simulink model "Regulacia_JCBM_Uloha3_S"  (R2022b)
settings: Solver=VariableStepAuto  StartTime=0.0  StopTime=4  RelTol=1e-8
values from neighbouring files (symbols this model uses):
  cfi = (Ua-Ra*IN)/wN    (= 2.66063720525)    [Regulacia_JCBM_M.m]
  h1 = double(h(1))    [Regulacia_JCBM_M.m]
  h2 = double(h(2))    [Regulacia_JCBM_M.m]
  Jc = Jm*8    (= 2.32)    [Regulacia_JCBM_M.m]
  Ki_2 = double(Ki_2)    [Regulacia_JCBM_M.m]
  Ki_5 = double(Ki_5)    [Regulacia_JCBM_M.m]
  La = 0.0081    [Regulacia_JCBM_M.m]
  Mz = MN    (= 132)    [Regulacia_JCBM_M.m]
  r1_2 = double(r1_2)    [Regulacia_JCBM_M.m]
  r1_5 = double(r1_5)    [Regulacia_JCBM_M.m]
  r2_2 = double(r2_2)    [Regulacia_JCBM_M.m]
  r2_5 = double(r2_5)    [Regulacia_JCBM_M.m]
  Ra = 0.522    [Regulacia_JCBM_M.m]
settings Model: Creator=hwswi  LastModifiedBy=hwswi

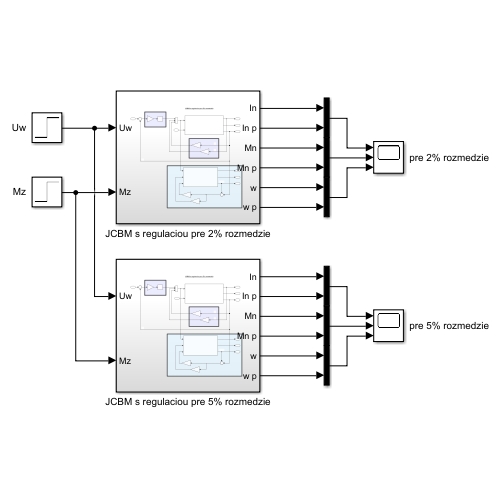
[thumbnail: Simulink's stored preview of the top-level diagram]
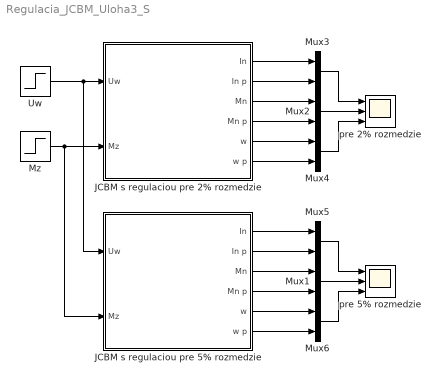
== system Regulacia_JCBM_Uloha3_S ==
  JCBM s regulaciou pre 2% rozmedzie : Subsystem
  JCBM s regulaciou pre 5% rozmedzie : Subsystem
  Mux{1..6} (6 alike) : Mux  Inputs=2
  Mz : Step  Time=2  After=Mz  SampleTime=0
  Uw : Step  Time=0  After=100  SampleTime=0
  pre 2% rozmedzie : Scope  NumInputPorts=3
  pre 5% rozmedzie : Scope  NumInputPorts=3
  wires:
  Uw/1 -> JCBM s regulaciou pre 5% rozmedzie/1(Uw), JCBM s regulaciou pre 2% rozmedzie/1(Uw)
  JCBM s regulaciou pre 2% rozmedzie/1(In) -> Mux3/1
  JCBM s regulaciou pre 2% rozmedzie/2(In p) -> Mux3/2
  JCBM s regulaciou pre 2% rozmedzie/4(Mn p) -> Mux2/2
  JCBM s regulaciou pre 2% rozmedzie/3(Mn) -> Mux2/1
  JCBM s regulaciou pre 2% rozmedzie/6(w p) -> Mux4/2
  JCBM s regulaciou pre 2% rozmedzie/5(w) -> Mux4/1
  JCBM s regulaciou pre 5% rozmedzie/5(w) -> Mux6/1
  JCBM s regulaciou pre 5% rozmedzie/6(w p) -> Mux6/2
  JCBM s regulaciou pre 5% rozmedzie/3(Mn) -> Mux1/1
  JCBM s regulaciou pre 5% rozmedzie/4(Mn p) -> Mux1/2
  JCBM s regulaciou pre 5% rozmedzie/2(In p) -> Mux5/2
  JCBM s regulaciou pre 5% rozmedzie/1(In) -> Mux5/1
  Mux4/1 -> pre 2% rozmedzie/3
  Mux6/1 -> pre 5% rozmedzie/3
  Mux2/1 -> pre 2% rozmedzie/2
  Mux1/1 -> pre 5% rozmedzie/2
  Mux5/1 -> pre 5% rozmedzie/1
  Mux3/1 -> pre 2% rozmedzie/1
  Mz/1 -> JCBM s regulaciou pre 5% rozmedzie/2(Mz), JCBM s regulaciou pre 2% rozmedzie/2(Mz)

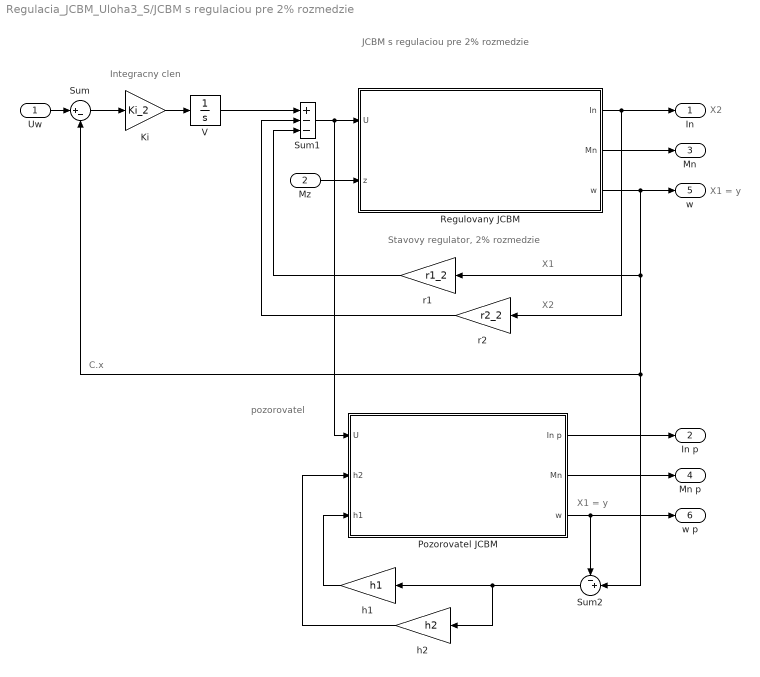
== system Regulacia_JCBM_Uloha3_S/JCBM s regulaciou pre 2% rozmedzie ==
  note: pozorovatel
  note: X1 = y
  note: X1 = y
  note: Stavovy regulator, 2% rozmedzie
  note: X2
  note: X1
  note: JCBM s regulaciou pre 2% rozmedzie
  note: Integracny clen
  note: X2
  note: C.x
  Uw : Inport
  Mz : Inport  Port=2
  Ki : Gain  Gain=Ki_2
  Pozorovatel JCBM : Subsystem
  Regulovany JCBM : Subsystem
  Sum : Sum  Inputs=|+-
  Sum1 : Sum  Inputs=+--
  Sum2 : Sum  Inputs=-+|
  V : Integrator
  h1 : Gain  Gain=h1
  h2 : Gain  Gain=h2
  "r1 " : Gain  Gain=r1_2
  "r2 " : Gain  Gain=r2_2
  In : Outport
  In p : Outport  Port=2
  Mn : Outport  Port=3
  Mn p : Outport  Port=4
  w : Outport  Port=5
  w p : Outport  Port=6
  wires:
  Uw/1 -> Sum/1
  Pozorovatel JCBM/3(w) -> w p/1, Sum2/1
  "r1 "/1 -> Sum1/3
  Sum1/1 -> Pozorovatel JCBM/1(U), Regulovany JCBM/1(U)
  Sum2/1 -> h2/1, h1/1
  Regulovany JCBM/1(In) -> "r2 "/1, In/1
  Regulovany JCBM/3(w) -> w/1, Sum2/2, Sum/2, "r1 "/1
  Ki/1 -> V/1
  "r2 "/1 -> Sum1/2
  Sum/1 -> Ki/1
  V/1 -> Sum1/1
  h2/1 -> Pozorovatel JCBM/2(h2)
  h1/1 -> Pozorovatel JCBM/3(h1)
  Regulovany JCBM/2(Mn) -> Mn/1
  Pozorovatel JCBM/1(In p) -> In p/1
  Pozorovatel JCBM/2(Mn) -> Mn p/1
  Mz/1 -> Regulovany JCBM/2(z)

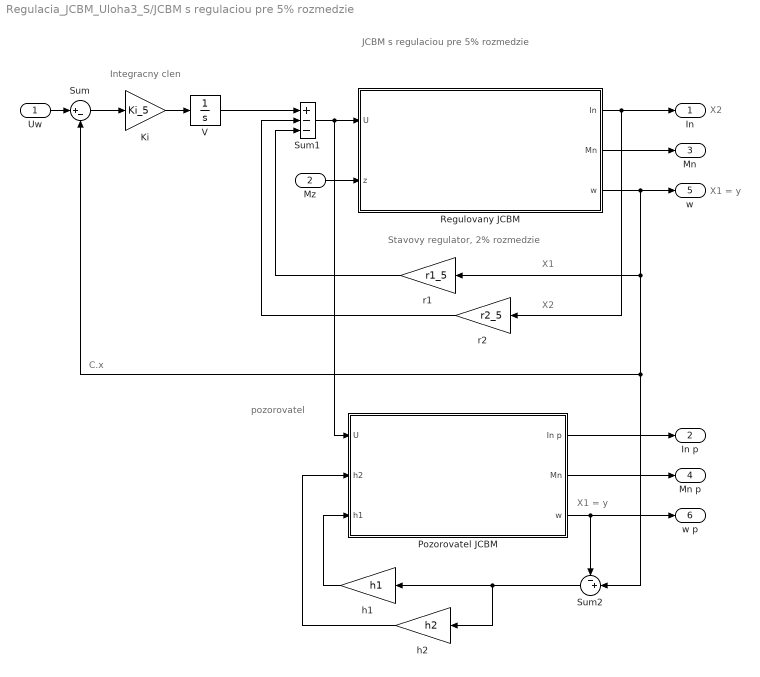
== system Regulacia_JCBM_Uloha3_S/JCBM s regulaciou pre 5% rozmedzie ==
  note: X1 = y
  note: pozorovatel
  note: X1
  note: Integracny clen
  note: JCBM s regulaciou pre 5% rozmedzie
  note: Stavovy regulator, 2% rozmedzie
  note: X2
  note: X2
  note: X1 = y
  note: C.x
  Uw : Inport
  Mz : Inport  Port=2
  Ki : Gain  Gain=Ki_5
  Pozorovatel JCBM : Subsystem
  Regulovany JCBM : Subsystem
  Sum : Sum  Inputs=|+-
  Sum1 : Sum  Inputs=+--
  Sum2 : Sum  Inputs=-+|
  V : Integrator
  h1 : Gain  Gain=h1
  h2 : Gain  Gain=h2
  "r1 " : Gain  Gain=r1_5
  "r2 " : Gain  Gain=r2_5
  In : Outport
  In p : Outport  Port=2
  Mn : Outport  Port=3
  Mn p : Outport  Port=4
  w : Outport  Port=5
  w p : Outport  Port=6
  wires:
  Regulovany JCBM/3(w) -> w/1, Sum2/2, Sum/2, "r1 "/1
  Regulovany JCBM/2(Mn) -> Mn/1
  "r1 "/1 -> Sum1/3
  V/1 -> Sum1/1
  Pozorovatel JCBM/1(In p) -> In p/1
  "r2 "/1 -> Sum1/2
  Ki/1 -> V/1
  Sum1/1 -> Pozorovatel JCBM/1(U), Regulovany JCBM/1(U)
  h2/1 -> Pozorovatel JCBM/2(h2)
  Pozorovatel JCBM/3(w) -> w p/1, Sum2/1
  Pozorovatel JCBM/2(Mn) -> Mn p/1
  h1/1 -> Pozorovatel JCBM/3(h1)
  Sum2/1 -> h2/1, h1/1
  Regulovany JCBM/1(In) -> "r2 "/1, In/1
  Sum/1 -> Ki/1
  Uw/1 -> Sum/1
  Mz/1 -> Regulovany JCBM/2(z)

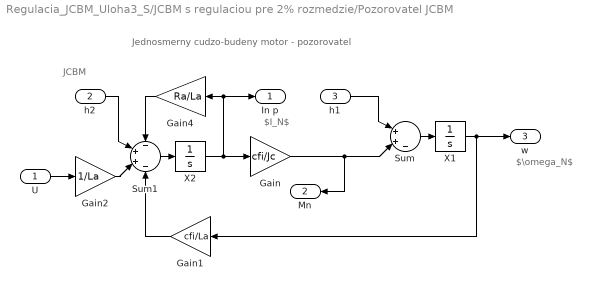
== system Regulacia_JCBM_Uloha3_S/JCBM s regulaciou pre 2% rozmedzie/Pozorovatel JCBM ==
  note: JCBM
  note: Jednosmerny cudzo-budeny motor - pozorovatel
  note: $\omega_N$
  note: $I_N$
  U : Inport
  h2 : Inport  Port=2
  h1 : Inport  Port=3
  Gain : Gain  Gain=cfi/Jc
  Gain1 : Gain  Gain=cfi/La
  Gain2 : Gain  Gain=1/La
  Gain4 : Gain  Gain=Ra/La
  Sum : Sum  Inputs=|++-
  Sum1 : Sum  Inputs=-++-
  X1 : Integrator
  X2 : Integrator
  In p : Outport
  Mn : Outport  Port=2
  w : Outport  Port=3
  wires:
  X1/1 -> Gain1/1, w/1
  X2/1 -> Gain/1, In p/1, Gain4/1
  Gain4/1 -> Sum1/1
  Sum1/1 -> X2/1
  Gain1/1 -> Sum1/4
  Sum/1 -> X1/1
  Gain2/1 -> Sum1/3
  U/1 -> Gain2/1
  h1/1 -> Sum/1
  h2/1 -> Sum1/2
  Gain/1 -> Mn/1, Sum/2

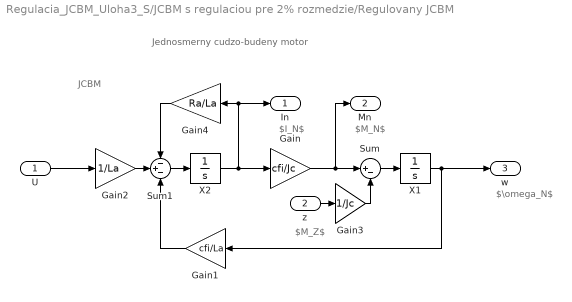
== system Regulacia_JCBM_Uloha3_S/JCBM s regulaciou pre 2% rozmedzie/Regulovany JCBM ==
  note: $M_N$
  note: $I_N$
  note: $\omega_N$
  note: Jednosmerny cudzo-budeny motor
  note: JCBM
  note: $M_Z$
  U : Inport
  z : Inport  Port=2
  Gain : Gain  Gain=cfi/Jc
  Gain1 : Gain  Gain=cfi/La
  Gain2 : Gain  Gain=1/La
  Gain3 : Gain  Gain=1/Jc
  Gain4 : Gain  Gain=Ra/La
  Sum : Sum  Inputs=|+-
  Sum1 : Sum  Inputs=-+-
  X1 : Integrator
  X2 : Integrator
  In : Outport
  Mn : Outport  Port=2
  w : Outport  Port=3
  wires:
  U/1 -> Gain2/1
  Gain2/1 -> Sum1/2
  Sum/1 -> X1/1
  Gain1/1 -> Sum1/3
  Sum1/1 -> X2/1
  Gain/1 -> Sum/1, Mn/1
  Gain4/1 -> Sum1/1
  X2/1 -> Gain/1, Gain4/1, In/1
  X1/1 -> Gain1/1, w/1
  Gain3/1 -> Sum/2
  z/1 -> Gain3/1

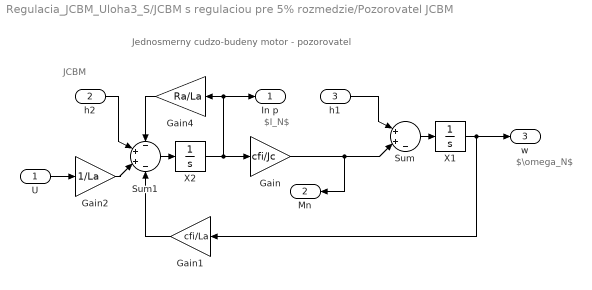
== system Regulacia_JCBM_Uloha3_S/JCBM s regulaciou pre 5% rozmedzie/Pozorovatel JCBM ==
  note: JCBM
  note: Jednosmerny cudzo-budeny motor - pozorovatel
  note: $\omega_N$
  note: $I_N$
  U : Inport
  h2 : Inport  Port=2
  h1 : Inport  Port=3
  Gain : Gain  Gain=cfi/Jc
  Gain1 : Gain  Gain=cfi/La
  Gain2 : Gain  Gain=1/La
  Gain4 : Gain  Gain=Ra/La
  Sum : Sum  Inputs=|++-
  Sum1 : Sum  Inputs=-++-
  X1 : Integrator
  X2 : Integrator
  In p : Outport
  Mn : Outport  Port=2
  w : Outport  Port=3
  wires:
  X1/1 -> Gain1/1, w/1
  X2/1 -> Gain/1, In p/1, Gain4/1
  Gain4/1 -> Sum1/1
  Sum1/1 -> X2/1
  Gain1/1 -> Sum1/4
  Sum/1 -> X1/1
  Gain2/1 -> Sum1/3
  U/1 -> Gain2/1
  h1/1 -> Sum/1
  h2/1 -> Sum1/2
  Gain/1 -> Mn/1, Sum/2

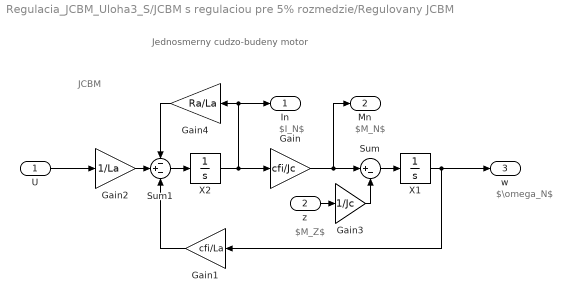
== system Regulacia_JCBM_Uloha3_S/JCBM s regulaciou pre 5% rozmedzie/Regulovany JCBM ==
  note: $M_N$
  note: $I_N$
  note: $\omega_N$
  note: Jednosmerny cudzo-budeny motor
  note: JCBM
  note: $M_Z$
  U : Inport
  z : Inport  Port=2
  Gain : Gain  Gain=cfi/Jc
  Gain1 : Gain  Gain=cfi/La
  Gain2 : Gain  Gain=1/La
  Gain3 : Gain  Gain=1/Jc
  Gain4 : Gain  Gain=Ra/La
  Sum : Sum  Inputs=|+-
  Sum1 : Sum  Inputs=-+-
  X1 : Integrator
  X2 : Integrator
  In : Outport
  Mn : Outport  Port=2
  w : Outport  Port=3
  wires:
  U/1 -> Gain2/1
  Gain2/1 -> Sum1/2
  Sum/1 -> X1/1
  Gain1/1 -> Sum1/3
  Sum1/1 -> X2/1
  Gain/1 -> Sum/1, Mn/1
  Gain4/1 -> Sum1/1
  X2/1 -> Gain/1, Gain4/1, In/1
  X1/1 -> Gain1/1, w/1
  z/1 -> Gain3/1
  Gain3/1 -> Sum/2
